simulink model "DFIG_WT_MPC"  (R2018a)
settings: Solver=VariableStepAuto  StartTime=0.0  StopTime=10.0  RelTol=1e-3
undefined symbols (not defined in the file): D1, Delta, powergui
libraries: powerlib x20, powerlib_meascontrol x18, fl_lib x6, nesl_utility x3, sdl_lib x1, simulink x1, re_lib x1
settings Model: Creator=Consultotal  LastModifiedBy=Consultotal
settings DebuggingCC: LibraryContextMissingDiagnostic=warning
settings SFSimCC: SimUseLocalCustomCode=on
settings RTWCC: RTWUseLocalCustomCode=on

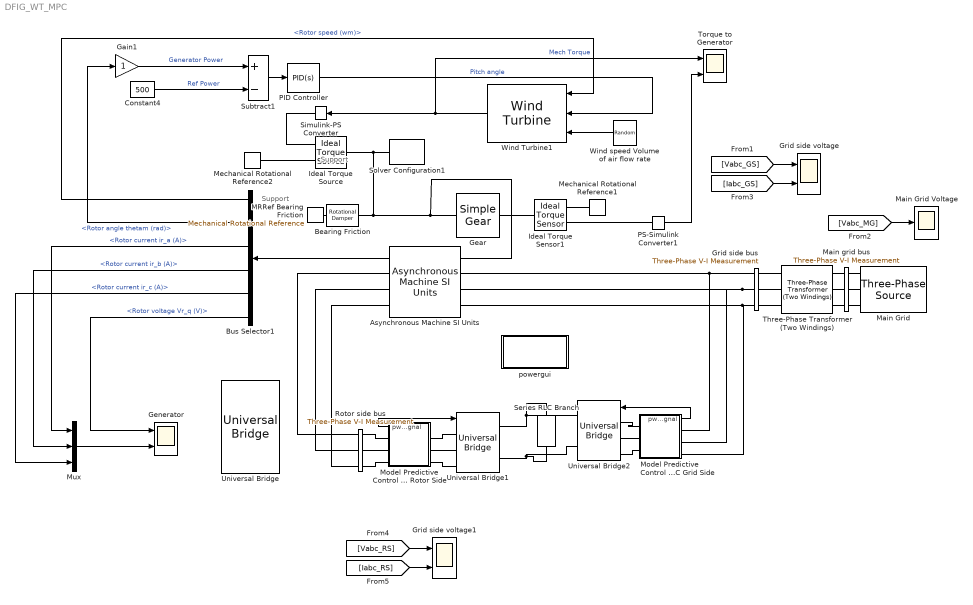
== system DFIG_WT_MPC ==
  note: Support
  note: Support
  Asynchronous Machine SI Units : powerlib/Machines/Asynchronous Machine SI Units  RotorType=Wound  PresetModel=No  MechanicalLoad=Mechanical rotational port  ShowDetailedParameters=on  ReferenceFrame=Synchronous  Units=SI  MeasurementBus=off  NominalParameters=[750e3 220 50]  Stator=[0.5968 0.0003495]  Rotor=[0.6258 0.005473]  Cage1=[0.4155 0.002066]  Cage2=[0.4168 0.0003495]  Lm=0.0354  Mechanical=[0.05 0.005879 2]  PolePairs=2  InitialConditions=[0 0 0 0 0 0 0 0]  SimulateSaturation=off  Saturation=[14.03593122, 27.81365428, 53.79336849, 72.68890987, 97.98006896, 148.6815601, 215.7428561, 302.9841135, 428.7778367 ; 230, 322, 414, 460, 506, 552, 598, 644, 690]  LoadFlowParameters=1492000  TsPowergui=0  TsBlock=-1  IterativeModel=Trapezoidal non iterative  IterativeDiscreteModel=Trapezoidal non iterative  Pmec=1.492e+006
  Bearing Friction : fl_lib/Mechanical/Rotational Elements/Rotational Damper  D=0.002 N*m/(rad/s)  w_specify=off  w_priority=High  w=0 rad/s  w_nominal_specify=off  w_nominal_unit=rad/s  w_nominal_value=1  t_specify=off  t_priority=High  t=0 N*m  t_nominal_specify=off  t_nominal_unit=N*m  t_nominal_value=1
  Bus Selector1 : BusSelector  OutputSignals=Mechanical.Rotor speed (wm),Mechanical.Rotor angle thetam (rad),Rotor measurements.Rotor current ir_a (A),Rotor measurements.Rotor current ir_b (A),Rotor measurements.Rotor current ir_c (A),Rotor measurements.Rotor voltage Vr_q (V)
  Constant4 : Constant  Value=500
  Gain1 : Gain
  Gear : sdl_lib/Gears/Simple Gear  ratio=40  rotation_direction=1  friction_model=1  T_noload=0.01 N*m  T_nom=0.2 N*m  efficiency_nom=0.8  efficiency=0.8  mu_visc=[ 0 0 ] N*m/(rad/s)  w_thr=0.01 rad/s  pwr_thr=0.001 W  enable_faults=0  efficiency_fault=0.05  external_fault=simscape.enum.onoff.off  temporal_fault=0  fault_time=5 s  fault_angles=pi / 12 rad  report_fault=1  temperature_TLU=[ 280 300 320 ] K  load_TLU=[ 1 5 10 ] N*m  efficiency_TLU=[ 0.95 0.9 0.85 ]  efficiency_TLU2=[ 0.85 0.8 0.75; 0.95 0.9 0.85; 0.85 0.8 0.7 ]  thermal_mass=50 J/K  T_init=300 K
      settings: SourceProductName=Simscape Driveline
  Generator : Scope  NumInputPorts=2
  Grid side bus : powerlib/Measurements/Three-Phase V-I Measurement  VoltageMeasurement=phase-to-phase  SetLabelV=on  LabelV=Vabc_GS  Vpu=off  VpuLL=off  CurrentMeasurement=yes  SetLabelI=on  LabelI=Iabc_GS  Ipu=off  Pbase=100e6  Vbase=18e3  OutputType=Complex  PhasorSimulation=off  PSBequivalent=0
  Grid side voltage : Scope  NumInputPorts=2
  Grid side voltage1 : Scope  NumInputPorts=2
  Ideal Torque Sensor1 : fl_lib/Mechanical/Mechanical Sensors/Ideal Torque Sensor
  Ideal Torque Source : fl_lib/Mechanical/Mechanical Sources/Ideal Torque Source
  MRRef Bearing Friction : fl_lib/Mechanical/Rotational Elements/Mechanical Rotational Reference
  Main grid bus : powerlib/Measurements/Three-Phase V-I Measurement  VoltageMeasurement=phase-to-phase  SetLabelV=on  LabelV=Vabc_MG  Vpu=off  VpuLL=off  CurrentMeasurement=no  SetLabelI=on  LabelI=Iabc_ld  Ipu=off  Pbase=100e6  Vbase=18e3  OutputType=Complex  PhasorSimulation=off  PSBequivalent=0
  Main Grid : powerlib/Electrical Sources/Three-Phase Source  InternalConnection=Yg  VoltagePhases=off  Voltage=34.5e3  PhaseAngle=0  Voltage_phases=[25e3 25e3 25e3]/sqrt(3)  PhaseAngles_phases=[0 -120 +120]  Frequency=50  NonIdealSource=on  SpecifyImpedance=off  Resistance=0.8929  Inductance=16.58e-3  ShortCircuitLevel=100e6  BaseVoltage=25e3  XRratio=7  BusType=swing  Pref=10e3  Qref=0  Prefabc=[10e3, 10e3, 10e3]  Qrefabc=[0, 0, 0]  Qmin=-inf  Qmax=inf
  Main Grid Voltage : Scope
  Mechanical Rotational Reference1 : fl_lib/Mechanical/Rotational Elements/Mechanical Rotational Reference
  Mechanical Rotational Reference2 : fl_lib/Mechanical/Rotational Elements/Mechanical Rotational Reference
  Model Predictive Control MPC Grid Side : Subsystem
  Model Predictive Control MPC Rotor Side : Subsystem
  Mux : Mux  Inputs=3
  PID Controller : simulink/Continuous/PID Controller  Controller=PID  Form=Parallel  TimeDomain=Continuous-time  SampleTime=-1  IntegratorMethod=Forward Euler  FilterMethod=Forward Euler  ControllerParametersSource=internal  P=5  I=8  D=0  UseFilter=on  N=100  TunerSelectOption=Transfer Function Based (PID Tuner App)  InitialConditionSource=internal  InitialConditionForIntegrator=0  InitialConditionForFilter=0  DifferentiatorICPrevScaledInput=0  ExternalReset=none  TrackingMode=off  Kt=1  LimitOutput=off  UpperSaturationLimit=inf  LowerSaturationLimit=-inf  LinearizeAsGain=on  AntiWindupMode=none  Kb=1  POutMin=[]  POutMax=[]  IOutMin=[]  IOutMax=[]  DOutMin=[]  DOutMax=[]  NOutMin=[]  NOutMax=[]  SumOutMin=[]  SumOutMax=[]  SaturationOutMin=[]  SaturationOutMax=[]  PParamMin=[]  PParamMax=[]  IParamMin=[]  IParamMax=[]  DParamMin=[]  DParamMax=[]  NParamMin=[]  NParamMax=[]  KbParamMin=[]  KbParamMax=[]  KtParamMin=[]  KtParamMax=[]  KbOutMin=[]  KbOutMax=[]  KtOutMin=[]  KtOutMax=[]  IntegratorOutMin=[]  IntegratorOutMax=[]  FilterOutMin=[]  FilterOutMax=[]  SumI1OutMin=[]  SumI1OutMax=[]  SumI2OutMin=[]  SumI2OutMax=[]  SumI3OutMin=[]  SumI3OutMax=[]  SumDOutMin=[]  SumDOutMax=[]  DifferentiatorOutMin=[]  DifferentiatorOutMax=[]  FilterDiffOutCoefMin=[]  FilterDiffOutCoefMax=[]  ReciprocalOutMin=[]  ReciprocalOutMax=[]  SumDenOutMin=[]  SumDenOutMax=[]  SumNumOutMin=[]  SumNumOutMax=[]  DivideOutMin=[]  DivideOutMax=[]  IntegratorContinuousStateAttributes=''  IntegratorStateMustResolveToSignalObject=off  IntegratorRTWStateStorageClass=Auto  FilterContinuousStateAttributes=''  FilterStateMustResolveToSignalObject=off  FilterRTWStateStorageClass=Auto
  PS-Simulink Converter1 : nesl_utility/PS-Simulink Converter  PhysicalDomain=network_engine_domain  SubClassName=ps_output  LeftPortType=input  RightPortType=output  PseudoPeriodic=off  Frequencies=[]  Unit=1  AffineConversion=off
  Rotor side bus : powerlib/Measurements/Three-Phase V-I Measurement  VoltageMeasurement=phase-to-phase  SetLabelV=on  LabelV=Vabc_RS  Vpu=off  VpuLL=off  CurrentMeasurement=yes  SetLabelI=on  LabelI=Iabc_RS  Ipu=off  Pbase=100e6  Vbase=18e3  OutputType=Complex  PhasorSimulation=off  PSBequivalent=0
  Series RLC Branch : powerlib/Elements/Series RLC Branch  LConnTagsString=__new0  RConnTagsString=__new0  BranchType=C  Resistance=1  Inductance=1e-3  SetiL0=off  InitialCurrent=0  Capacitance=1e6  Setx0=off  InitialVoltage=0  Measurements=None
  Simulink-PS Converter : nesl_utility/Simulink-PS Converter  PhysicalDomain=network_engine_domain  SubClassName=ps_input  LeftPortType=input  RightPortType=output  PseudoPeriodic=off  Frequencies=[]  NoiseDistribution=none  NoiseParameters=[]  Unit=1  AffineConversion=off  FilteringAndDerivatives=provide  SimscapeFilterOrder=1  InputFilterTimeConstant=0.001  UdotUserProvided=0
  Solver Configuration1 : nesl_utility/Solver Configuration  PhysicalDomain=network_engine_domain  SubClassName=solver  LeftPortType=input  RightPortType=generic  Tones=[]  Harmonics=[]  SimulateNoise=off  Profile=off  UseLocalSampling=off  EnableSwitchedLinearOptims=on  FrequencyDomain=off  UseCCode=off  RelTol=0.001  AbsTol=1e-06  MinStep=1e-09  ToWorkspace=off  RevertToSquareIcSolve=off  NumHomotopyIterations=100  PhasorMode=off  PhasorModeNumHarmonics=1  DoDC=off  ResidualTolerance=1e-9  UseLocalSolver=on  LocalSolverChoice=NE_BACKWARD_EULER_ADVANCER  LocalSolverSampleTime=.001  DoFixedCost=on  MaxNonlinIter=3  MaxModeIter=2  LinearAlgebra=Sparse  EquationFormulation=NE_TIME_EF  DelaysMemoryBudget=1024  AutomaticFiltering=on  FilteringTimeConstant=0.001  PartitionStorageMethod=AS_NEEDED  PartitionMemoryBudget=1024
  Subtract1 : Sum  Inputs=+-
  Three-Phase Transformer (Two Windings) : powerlib/Elements/Three-Phase Transformer (Two Windings)  Winding1Connection=Yg  Winding2Connection=Delta (D1)  CoreType=Three single-phase transformers  SetSaturation=off  Hysteresis=off  DataFile='hysteresis'  SetInitialFlux=off  Measurements=None  UNITS=pu  NominalPower=[ 75e3 , 50 ]  Winding1=[ 220 , 0.002 , 0.08 ]  Winding2=[ 34.5e3 , 0.002 , 0.08 ]  Rm=1e4  Lm=1e4  L0=0.5  Saturation=[ 0,0 ; 0.0024,1.2 ; 1.0,1.52 ]  InitialFluxes=[ 0.8 , -0.8 , 0.7 ]  MoreParameters=off  BreakLoop=off  DataType=off  TransfoNumber=1
  "Torque to Generator " : Scope  NumInputPorts=2
  Universal Bridge : powerlib/Power Electronics/Universal Bridge  Arms=3  SnubberResistance=1e5  SnubberCapacitance=inf  Device=Thyristors  Ron=1e-3  Lon=0  ForwardVoltages="[  0  0  ]"  ForwardVoltage=0  GTOparameters=[ 10e-6 , 20e-6 ]  IGBTparameters=[ 1e-6 , 2e-6 ]  Measurements=None  Measurements_2=None  converterType=Rectifier
  Universal Bridge1 : powerlib/Power Electronics/Universal Bridge  Arms=3  SnubberResistance=1e5  SnubberCapacitance=inf  Device=MOSFET / Diodes  Ron=1e-3  Lon=0  ForwardVoltages="[  0  0  ]"  ForwardVoltage=0  GTOparameters=[ 10e-6 , 20e-6 ]  IGBTparameters=[ 1e-6 , 2e-6 ]  Measurements=None  Measurements_2=None  converterType=Rectifier
  Universal Bridge2 : powerlib/Power Electronics/Universal Bridge  Arms=3  SnubberResistance=1e5  SnubberCapacitance=inf  Device=MOSFET / Diodes  Ron=1e-3  Lon=0  ForwardVoltages="[  0  0  ]"  ForwardVoltage=0  GTOparameters=[ 10e-6 , 20e-6 ]  IGBTparameters=[ 1e-6 , 2e-6 ]  Measurements=None  Measurements_2=None  converterType=Rectifier
  Wind Turbine1 : re_lib/Wind Generation/Wind Turbine  Pnom=1.5e6  Pelec_base=1.5e6/0.9  wind_base=12  P_wind_base=0.73  speed_nom=1.2  pitch_angle=0  c1_c6="[0.51763          116          0.4            5           21     0.006795]"  cp_nom=0.48  lambda_nom=8.1
      settings: SourceProductName=Simscape Power Systems  SourceProductBaseCode=PS
  Wind speed Volume of air flow rate : UniformRandomNumber  Minimum=2  Maximum=9  Seed=14  SampleTime=0.001
  powergui : Subsystem  Priority=1  AncestorBlock=powerlib/powergui  DialogController=POWERSYS.PowerSysDialog  InitFcn=powergui( 'InitFcn_Callback' , gcb , 0 , [ ] );  mask(PSB option menu block){SimulationMode=Discrete, SampleTime=50e-6, frequency=60, Iterations=50, frequencyindice=0, Pbase=100e6, ErrMax=1e-4, UnitsV=kV, UnitsW=MW, buscounter=0, FunctionMessages=off, echomessages=off, EnableUseOfTLC=off, CurrentSourceSwitches=off, DisableSnubberDevices=off, DisableRonSwitches=off, DisableVfSwitches=off, DisplayEquations=off, SolverType=Tustin/Backward Euler (TBE), Interpol=off, ExternalGateDelay=off, methode=off, Ts=100, x0status=blocks, SPID=on, SwTol=0, HookPort=off, RestoreLinks=warning, ResistiveCurrentMeasurement=off, Frange=[0:2:500], Ylog=off, Xlog=on, ShowGrid=off, save=off, variable=ZData, structure=0, ZoomFFT=off, StartTime=0.0, cycles=1, DisplayStyle=1, fundamental=60, FreqAxis=off, MaxFrequency=1000, frequencyindicesteady=1, RmsSteady=1, display=off}
      mask prompts: SimulationMode "Simulation type:"; SampleTime "Sample time (s):"; frequency "Frequency (Hz):"; Iterations "Max iterations"; frequencyindice "Frequency (Hz)"; Pbase "Base power (VA)"; ErrMax "PQ tolerance (pu)"; UnitsV "Voltage units"; UnitsW "Power units"; buscounter "Load flow bus counter"; FunctionMessages "Disable Specialized Power Systems warnings"; echomessages "Display Specialized Power Systems compilation messages"; EnableUseOfTLC "Use TLC file when in Accelerator Simulation Mode and for code generation"; CurrentSourceSwitches "Disable ideal switching"; DisableSnubberDevices "Disable snubbers in switching devices"; DisableRonSwitches "Disable Ron resistances in switching devices"; DisableVfSwitches "Disable forward voltages in switching devices"; DisplayEquations "Display circuit differential equations"; SolverType "Discrete solver"; Interpol "Interpolate switching events"; ExternalGateDelay "Use time-stamped gate signals"; methode "Store switching topologies"; Ts "Buffer size (MBytes):"; x0status "Start simulation with initial electrical states from:"; SPID "Use ideal switching devices"; SwTol "Switch tolerance"; HookPort "Allow multiple powergui blocks"; RestoreLinks "Restore disabled links of Simscape Power Systems ST blocks:"; ResistiveCurrentMeasurement "Use non ideal current measurement blocks (1e-4Ohm internal resistance)"; Frange "Frequency Range"; Ylog "Log impedance"; Xlog "log Frequency"; ShowGrid "grid"; save "Save Data To Workspace"; variable "Variable Name"; structure "Structure Name (PSBFFTSCOPE)"; ZoomFFT "ZoomFFT (PSBFFTSCOPE)"; StartTime "Start Time (PSBFFTSCOPE)"; cycles "Cycles (PSBFFTSCOPE)"; DisplayStyle "Display style (PSBFFTSCOPE)"; fundamental "Fundamental (PSBFFTSCOPE)"; FreqAxis "Frequency Axis (PSBFFTSCOPE)"; MaxFrequency "Max Frequency (PSBFFTSCOPE)"; frequencyindicesteady "Frequency indice (STEADYSTATE)"; RmsSteady "RMS display (STEADYSTATE)"; display "Display Results"
      mask help: Set simulation type, simulation parameters, and preferences.
      mask init:
      | dispMessage = powergui('MaskInitialization',gcb,SimulationMode,SampleTime);
      settings: PreSaveFcn=powergui( 'PreSaveFcn_Callback' , gcb , [ ] , [ ] );  OpenFcn=sps_rtmsupport('OpenFcn',gcbh)
      mask Help: helpview(psbhelp)
      mask TypeOptions SimulationMode: Continuous | Discrete | Phasor
      mask Callback SimulationMode: powergui('SimulationType',[],[],gcb);
      mask TypeOptions UnitsV: V | kV
      mask TypeOptions UnitsW: W | kW | MW
      mask Callback CurrentSourceSwitches: powergui('SimulationType',[],[],gcb);
      mask TypeOptions SolverType: Tustin/Backward Euler (TBE) | Tustin | Backward Euler
      mask Callback SolverType: powergui('SimulationType',[],[],gcb);
      mask Callback Interpol: powergui('SimulationType',[],[],gcb);
      mask Callback ExternalGateDelay: powergui('SimulationType',[],[],gcb);
      mask Callback methode: powergui('SimulationType',[],[],gcb);
      mask TypeOptions x0status: blocks | steady | zero
      mask TypeOptions RestoreLinks: yes | warning | no
      mask Callback display: sps_rtmsupport('parametereditingmodes',gcbh) % Will be executed last in parameter callbacks to ensure mask enable consistency
      mask DialogControl SolverTab Prompt: Solver
      mask DialogControl AutoSolverNote Prompt: To enable the Powergui solver settings, unselect auto (Automatic solver selection) solver in the Simulink solver options.
      mask DialogControl AnalysisTools Prompt: Tools
      mask DialogControl SteadyState Prompt: Steady-State
      mask DialogControl SteadyState Callback: close_system(gcb); power_steadystate(bdroot(gcb),gcb);
      mask DialogControl InitialState Prompt: Initial State
      mask DialogControl InitialState Callback: close_system(gcb); power_initstates(bdroot(gcb),gcb)
      mask DialogControl MachineInitialization Prompt: Machine Initialization
      mask DialogControl MachineInitialization Callback: close_system(gcb); power_loadflow(bdroot(gcb),gcb);
      mask DialogControl ImpedanceMeasurement Prompt: Impedance Measurement
      mask DialogControl ImpedanceMeasurement Callback: close_system(gcb); power_zmeter(bdroot(gcb),gcb);
      mask DialogControl FFTAnalysis Prompt: FFT Analysis
      mask DialogControl FFTAnalysis Callback: close_system(gcb); power_fftscope(bdroot(gcb),gcb);
      mask DialogControl LinearSystemAnalyzer Prompt: Use Linear System Analyzer
      mask DialogControl LinearSystemAnalyzer Callback: close_system(gcb); power_ltiview(bdroot(gcb),gcb);
      mask DialogControl HysteresisDesign Prompt: Hysteresis Design
      mask DialogControl HysteresisDesign Callback: close_system(gcb); power_hysteresis(bdroot(gcb),gcb);
      mask DialogControl RLCLineParameters Prompt: RLC Line Parameters
      mask DialogControl RLCLineParameters Callback: close_system(gcb); power_lineparam(bdroot(gcb),gcb);
      mask DialogControl GenerateReprot Prompt: Generate Report
      mask DialogControl GenerateReprot Callback: close_system(gcb); power_report(bdroot(gcb),gcb);
      mask DialogControl Control14 Prompt: Customize SPS blocks
      mask DialogControl Control14 Callback: close_system(gcb); power_customize;
      mask DialogControl LoadFlow Prompt: Load Flow
      mask DialogControl LoadFlow Callback: close_system(gcb); power_loadflow('-v2',bdroot(gcb));
      mask DialogControl Container14 Prompt: Load flow settings
      mask DialogControl ParameterTabVar012 Prompt: Preferences
      mask Display: color('blue'),disp(dispMessage)
  wires:
  PID Controller/1 -> Wind Turbine1/2  "Pitch angle"
  Subtract1/1 -> PID Controller/1
  Bus Selector1/1 -> Wind Turbine1/1  "<Rotor speed (wm)>"
  Bus Selector1/2 -> Gain1/1  "<Rotor angle thetam (rad)>"
  Wind Turbine1/1 -> Simulink-PS Converter/1, "Torque to Generator "/1  "Mech Torque"
  Constant4/1 -> Subtract1/2  "Ref Power"
  Gain1/1 -> Subtract1/1  "Generator Power"
  Wind speed Volume of air flow rate/1 -> Wind Turbine1/3
  Asynchronous Machine SI Units/1 -> Bus Selector1/1
  PS-Simulink Converter1/1 -> "Torque to Generator "/2
  Bus Selector1/6 -> Generator/1  "<Rotor voltage Vr_q (V)>"
  [Vabc_GS] -> Grid side voltage/1
  [Vabc_MG] -> Main Grid Voltage/1
  Mux/1 -> Generator/2
  Bus Selector1/3 -> Mux/1  "<Rotor current ir_a (A)>"
  Bus Selector1/4 -> Mux/2  "<Rotor current ir_b (A)>"
  Bus Selector1/5 -> Mux/3  "<Rotor current ir_c (A)>"
  Model Predictive Control MPC Grid Side/1(pwm signal) -> Universal Bridge2/1
  [Iabc_GS] -> Grid side voltage/2
  [Iabc_RS] -> Grid side voltage1/2
  [Vabc_RS] -> Grid side voltage1/1
  Model Predictive Control MPC Rotor Side/1(pwm signal) -> Universal Bridge1/1
  connections:
  Series RLC Branch/LConn1 -- Universal Bridge1/RConn1 -- Universal Bridge2/RConn1
  Series RLC Branch/RConn1 -- Universal Bridge2/RConn2 -- Universal Bridge1/RConn2
  Asynchronous Machine SI Units/RConn3 -- Rotor side bus/LConn3
  Ideal Torque Sensor1/LConn1 -- Gear/RConn1
  Mechanical Rotational Reference1/LConn1 -- Ideal Torque Sensor1/RConn1
  Ideal Torque Sensor1/RConn2 -- PS-Simulink Converter1/LConn1
  Simulink-PS Converter/RConn1 -- Ideal Torque Source/RConn1
  Ideal Torque Source/RConn2 -- Mechanical Rotational Reference2/LConn1
  Gear/LConn1 -- Asynchronous Machine SI Units/LConn1 -- Ideal Torque Source/LConn1 -- Solver Configuration1/RConn1 -- Bearing Friction/LConn1
  Rotor side bus/LConn2 -- Asynchronous Machine SI Units/RConn2
  Rotor side bus/LConn1 -- Asynchronous Machine SI Units/RConn1
  MRRef Bearing Friction/LConn1 -- Bearing Friction/RConn1
  Main Grid/RConn1 -- Main grid bus/RConn1
  Main grid bus/RConn2 -- Main Grid/RConn2
  Main Grid/RConn3 -- Main grid bus/RConn3
  Three-Phase Transformer (Two Windings)/RConn3 -- Main grid bus/LConn3
  Three-Phase Transformer (Two Windings)/RConn2 -- Main grid bus/LConn2
  Three-Phase Transformer (Two Windings)/RConn1 -- Main grid bus/LConn1
  Model Predictive Control MPC Grid Side/RConn1 -- Asynchronous Machine SI Units/LConn2 -- Grid side bus/LConn1
  Grid side bus/LConn2 -- Asynchronous Machine SI Units/LConn3 -- Model Predictive Control MPC Grid Side/RConn2
  Model Predictive Control MPC Grid Side/RConn3 -- Asynchronous Machine SI Units/LConn4 -- Grid side bus/LConn3
  Three-Phase Transformer (Two Windings)/LConn1 -- Grid side bus/RConn1
  Three-Phase Transformer (Two Windings)/LConn2 -- Grid side bus/RConn2
  Three-Phase Transformer (Two Windings)/LConn3 -- Grid side bus/RConn3
  Universal Bridge2/LConn1 -- Model Predictive Control MPC Grid Side/LConn1
  Universal Bridge2/LConn2 -- Model Predictive Control MPC Grid Side/LConn2
  Universal Bridge2/LConn3 -- Model Predictive Control MPC Grid Side/LConn3
  Model Predictive Control MPC Rotor Side/LConn2 -- Universal Bridge1/LConn1
  Universal Bridge1/LConn2 -- Model Predictive Control MPC Rotor Side/LConn3
  Model Predictive Control MPC Rotor Side/LConn4 -- Universal Bridge1/LConn3
  Model Predictive Control MPC Rotor Side/RConn3 -- Rotor side bus/RConn3
  Rotor side bus/RConn2 -- Model Predictive Control MPC Rotor Side/RConn2
  Rotor side bus/RConn1 -- Model Predictive Control MPC Rotor Side/RConn1

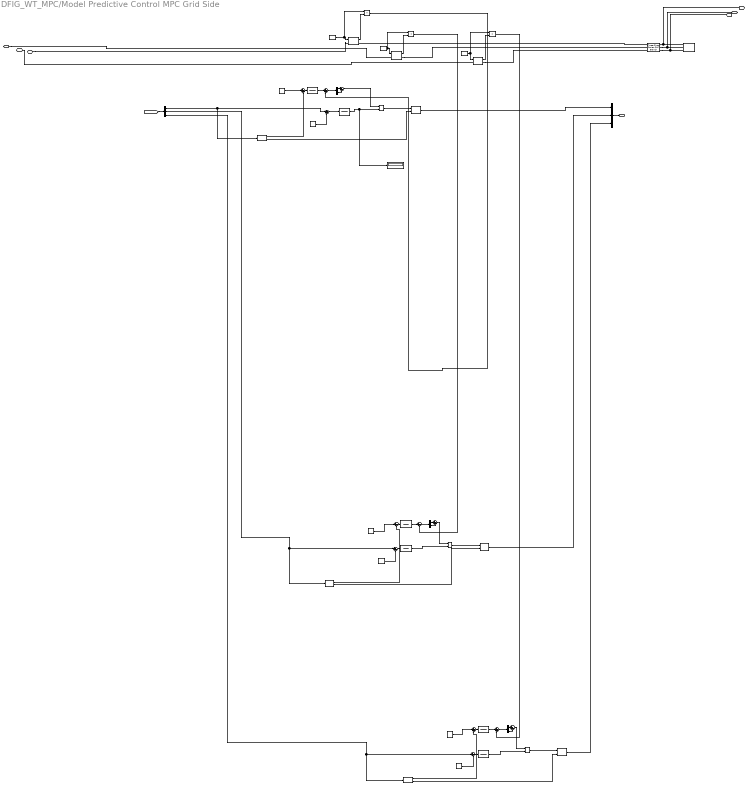
== system DFIG_WT_MPC/Model Predictive Control MPC Grid Side ==
  note: Amplitude of output voltage
  note: Delta ws
  note: deltaw
  note: wMG
  note: deltaE
  note: E*MG
  note: Fc= 50 Hz
  note: Amplitude of output voltage
  note: Delta ws
  note: deltaw
  note: wMG
  note: deltaE
  note: E*MG
  note: Fc= 50 Hz
  note: Amplitude of output voltage
  note: Delta ws
  note: deltaw
  note: wMG
  note: deltaE
  note: E*MG
  note: Fc= 50 Hz
  AC grid3 : powerlib/Elements/Three-Phase Series RLC Load  LConnTagsString=A|B|C  Configuration=Y (grounded)  NominalVoltage=240  Vabc=[1e3 1e3 1e3]  Vabcp=[1e3 1e3 1e3]  NominalFrequency=50  UnbalancedPower=off  ActivePower=10e4  InductivePower=0  CapacitivePower=0  Pabc=[10e3 9e3 11e3]  QLabc=[100 90 110]  QCabc=[100 90 110]  Pabcp=[10e3 9e3 11e3]  QLabcp=[100 90 110]  QCabcp=[100 90 110]  Measurements=None  LoadType=constant Z
  Demux : Demux  Outputs=3
  Demux1 : Demux  Outputs=2
  Demux3 : Demux  Outputs=2
  Demux4 : Demux  Outputs=2
  Discrete Transfer Fcn GE(S) : DiscreteTransferFcn  SampleTime=2e-6
  Discrete Transfer Fcn GE(S)1 : DiscreteTransferFcn  SampleTime=2e-6
  Discrete Transfer Fcn GE(S)2 : DiscreteTransferFcn  SampleTime=2e-6
  Discrete Transfer Fcn Gw(S) : DiscreteTransferFcn  SampleTime=2e-6
  Discrete Transfer Fcn Gw(S)1 : DiscreteTransferFcn  SampleTime=2e-6
  Discrete Transfer Fcn Gw(S)2 : DiscreteTransferFcn  SampleTime=2e-6
  Display1 : Display
  E*MG Amplitude's reference : Constant  Value=220
  E*MG Amplitude's reference1 : Constant  Value=220
  E*MG Amplitude's reference2 : Constant  Value=220
  Mux : Mux  Inputs=3
  PLL : powerlib_meascontrol/PLL/PLL  Fmin=45  Par_Init=[0, 50]  ParK=[0.45, 1.69, 0]  TcD=1e-4  MaxRateChangeFreq=12  FilterCutOffFreq=25  Ts=2e-6  AGC=on
      settings: SourceProductName=Simscape Power Systems  SourceProductBaseCode=PS
  PLL1 : powerlib_meascontrol/PLL/PLL  Fmin=45  Par_Init=[0, 50]  ParK=[0.45, 1.69, 0]  TcD=1e-4  MaxRateChangeFreq=12  FilterCutOffFreq=25  Ts=2e-6  AGC=on
      settings: SourceProductName=Simscape Power Systems  SourceProductBaseCode=PS
  PLL2 : powerlib_meascontrol/PLL/PLL  Fmin=45  Par_Init=[0, 50]  ParK=[0.45, 1.69, 0]  TcD=1e-4  MaxRateChangeFreq=12  FilterCutOffFreq=25  Ts=2e-6  AGC=on
      settings: SourceProductName=Simscape Power Systems  SourceProductBaseCode=PS
  PWM Generator (2-Level) : powerlib_meascontrol/Pulse & Signal Generators/PWM Generator (2-Level)  ModulatorType=Single-phase half-bridge (2 pulses)  ModulatorMode=Synchronized  Fc=27*50  Pc=90  nF=1  MinMax="[ -1  1 ]"  SamplingTechnique=Natural  ModulatingSignals=off  m=0.8  Freq=60  Phase=0  Ts=0  ShowCarrierOutport=off
      settings: SourceProductName=Simscape Power Systems
  PWM Generator (2-Level)1 : powerlib_meascontrol/Pulse & Signal Generators/PWM Generator (2-Level)  ModulatorType=Single-phase half-bridge (2 pulses)  ModulatorMode=Synchronized  Fc=27*50  Pc=90  nF=1  MinMax="[ -1  1 ]"  SamplingTechnique=Natural  ModulatingSignals=off  m=0.8  Freq=60  Phase=0  Ts=0  ShowCarrierOutport=off
      settings: SourceProductName=Simscape Power Systems
  PWM Generator (2-Level)2 : powerlib_meascontrol/Pulse & Signal Generators/PWM Generator (2-Level)  ModulatorType=Single-phase half-bridge (2 pulses)  ModulatorMode=Synchronized  Fc=27*50  Pc=90  nF=1  MinMax="[ -1  1 ]"  SamplingTechnique=Natural  ModulatingSignals=off  m=0.8  Freq=60  Phase=0  Ts=0  ShowCarrierOutport=off
      settings: SourceProductName=Simscape Power Systems
  Plant1 : powerlib/Elements/Three-Phase Series RLC Branch  LConnTagsString=A|B|C  RConnTagsString=A|B|C  BranchType=R  Resistance=0.05  Inductance=0.0002  Capacitance=0  Measurements=None
  Product1 : Product
  Product2 : Product
  Product3 : Product
  Product5 : Product  SampleTime=0  RndMeth=Zero
  Product7 : Product  SampleTime=0  RndMeth=Zero
  Product9 : Product  SampleTime=0  RndMeth=Zero
  Stair Generator : powerlib_meascontrol/Pulse & Signal Generators/Stair Generator  t="[0 3/60  8.25/60 ]"  e=[1 0 1]  Ts=0
      settings: SourceProductName=Simscape Power Systems
  Stair Generator1 : powerlib_meascontrol/Pulse & Signal Generators/Stair Generator  t="[0 3/60  8.25/60 ]"  e=[1 0 1]  Ts=0
      settings: SourceProductName=Simscape Power Systems
  Stair Generator2 : powerlib_meascontrol/Pulse & Signal Generators/Stair Generator  t="[0 3/60  8.25/60 ]"  e=[1 0 1]  Ts=0
      settings: SourceProductName=Simscape Power Systems
  Sum{4..6,9,11..13,16,19..21,24} (12 alike) : Sum  Inputs=|+-
  bypass : powerlib/Power Electronics/Ideal Switch  Ron=0.001  Lon=0  IC=0  Rs=1e5  Cs=inf  Measurements=on
  bypass1 : powerlib/Power Electronics/Ideal Switch  Ron=0.001  Lon=0  IC=0  Rs=1e5  Cs=inf  Measurements=on
  bypass2 : powerlib/Power Electronics/Ideal Switch  Ron=0.001  Lon=0  IC=0  Rs=1e5  Cs=inf  Measurements=on
  wi* island Frequency's reference : Constant  Value=50
  wi* island Frequency's reference1 : Constant  Value=50
  wi* island Frequency's reference2 : Constant  Value=50
  a : PMIOPort  Side=Right
  b : PMIOPort  Port=2  Side=Right
  c : PMIOPort  Port=3  Side=Right
  A : PMIOPort  Port=4  Side=Left
  B : PMIOPort  Port=5  Side=Left
  C : PMIOPort  Port=6  Side=Left
  pwm signal : Outport
  wires:
  Sum4/1 -> Discrete Transfer Fcn Gw(S)/1
  PLL1/2 -> PWM Generator (2-Level)1/2
  Discrete Transfer Fcn Gw(S)2/1 -> Sum20/1
  Demux/2 -> PLL1/1, Sum13/1
  Demux/3 -> PLL/1, Sum6/1
  bypass2/1 -> Product3/2
  Sum9/1 -> Product5/1
  Sum12/1 -> Demux3/1
  Sum11/1 -> Discrete Transfer Fcn Gw(S)1/1
  Demux3/1 -> Sum16/1
  E*MG Amplitude's reference1/1 -> Sum13/2
  PWM Generator (2-Level)2/1 -> Mux/1
  PWM Generator (2-Level)/1 -> Mux/3
  E*MG Amplitude's reference/1 -> Sum6/2
  PLL/2 -> PWM Generator (2-Level)/2
  Sum20/1 -> Demux4/1
  Stair Generator/1 -> bypass/1, Product2/1
  PLL2/1 -> Sum19/2
  wi* island Frequency's reference1/1 -> Sum11/1
  Stair Generator1/1 -> bypass1/1, Product1/1
  Discrete Transfer Fcn GE(S)1/1 -> Product7/2
  PLL2/2 -> PWM Generator (2-Level)2/2
  Product1/1 -> Sum12/2
  PLL1/1 -> Sum11/2
  E*MG Amplitude's reference2/1 -> Sum21/2
  Demux3/2 -> Sum16/2
  Product9/1 -> PWM Generator (2-Level)2/1
  Sum24/1 -> Product9/1
  Discrete Transfer Fcn Gw(S)/1 -> Sum5/1
  Product3/1 -> Sum5/2
  Discrete Transfer Fcn GE(S)2/1 -> Display1/1, Product9/2
  wi* island Frequency's reference2/1 -> Sum19/1
  Demux4/1 -> Sum24/1
  bypass/1 -> Product2/2
  Demux1/1 -> Sum9/1
  wi* island Frequency's reference/1 -> Sum4/1
  Sum19/1 -> Discrete Transfer Fcn Gw(S)2/1
  Demux1/2 -> Sum9/2
  bypass1/1 -> Product1/2
  Product2/1 -> Sum20/2
  Product5/1 -> PWM Generator (2-Level)/1
  Mux/1 -> pwm signal/1
  Sum6/1 -> Discrete Transfer Fcn GE(S)/1
  Discrete Transfer Fcn Gw(S)1/1 -> Sum12/1
  Sum13/1 -> Discrete Transfer Fcn GE(S)1/1
  Sum16/1 -> Product7/1
  PWM Generator (2-Level)1/1 -> Mux/2
  Demux4/2 -> Sum24/2
  Sum5/1 -> Demux1/1
  Discrete Transfer Fcn GE(S)/1 -> Product5/2
  Sum21/1 -> Discrete Transfer Fcn GE(S)2/1
  Demux/1 -> PLL2/1, Sum21/1
  Product7/1 -> PWM Generator (2-Level)1/1
  PLL/1 -> Sum4/2
  Stair Generator2/1 -> bypass2/1, Product3/1
  [Vabc_GS] -> Demux/1
  connections:
  C/RConn1 -- bypass/LConn1
  A/RConn1 -- bypass1/LConn1
  B/RConn1 -- bypass2/LConn1
  bypass2/RConn1 -- Plant1/RConn3
  bypass1/RConn1 -- Plant1/RConn2
  Plant1/RConn1 -- bypass/RConn1
  Plant1/LConn3 -- c/RConn1 -- AC grid3/LConn3
  Plant1/LConn2 -- b/RConn1 -- AC grid3/LConn2
  Plant1/LConn1 -- a/RConn1 -- AC grid3/LConn1

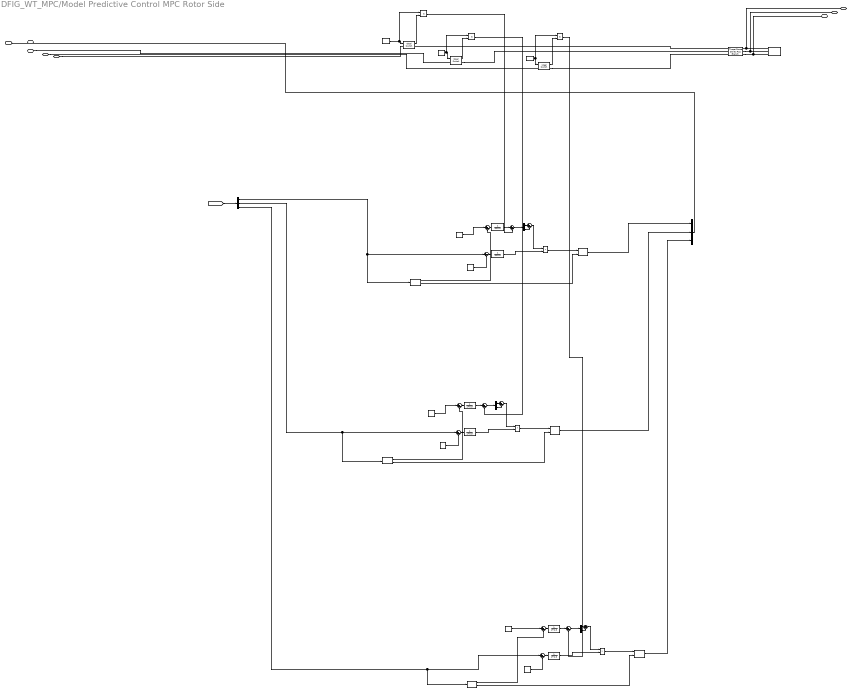
== system DFIG_WT_MPC/Model Predictive Control MPC Rotor Side ==
  note: Amplitude of output voltage
  note: Delta ws
  note: deltaw
  note: wMG
  note: deltaE
  note: E*MG
  note: Fc= 50 Hz
  note: Amplitude of output voltage
  note: Delta ws
  note: deltaw
  note: wMG
  note: deltaE
  note: E*MG
  note: Fc= 50 Hz
  note: Amplitude of output voltage
  note: Delta ws
  note: deltaw
  note: wMG
  note: deltaE
  note: E*MG
  note: Fc= 50 Hz
  AC grid3 : powerlib/Elements/Three-Phase Series RLC Load  LConnTagsString=A|B|C  Configuration=Y (grounded)  NominalVoltage=240  Vabc=[1e3 1e3 1e3]  Vabcp=[1e3 1e3 1e3]  NominalFrequency=50  UnbalancedPower=off  ActivePower=10e4  InductivePower=0  CapacitivePower=0  Pabc=[10e3 9e3 11e3]  QLabc=[100 90 110]  QCabc=[100 90 110]  Pabcp=[10e3 9e3 11e3]  QLabcp=[100 90 110]  QCabcp=[100 90 110]  Measurements=None  LoadType=constant Z
  Demux : Demux  Outputs=3
  Demux1 : Demux  Outputs=2
  Demux3 : Demux  Outputs=2
  Demux4 : Demux  Outputs=2
  Discrete Transfer Fcn GE(S) : DiscreteTransferFcn  SampleTime=2e-6
  Discrete Transfer Fcn GE(S)1 : DiscreteTransferFcn  SampleTime=2e-6
  Discrete Transfer Fcn GE(S)2 : DiscreteTransferFcn  SampleTime=2e-6
  Discrete Transfer Fcn Gw(S) : DiscreteTransferFcn  SampleTime=2e-6
  Discrete Transfer Fcn Gw(S)1 : DiscreteTransferFcn  SampleTime=2e-6
  Discrete Transfer Fcn Gw(S)2 : DiscreteTransferFcn  SampleTime=2e-6
  E*MG Amplitude's reference : Constant  Value=220
  E*MG Amplitude's reference1 : Constant  Value=220
  E*MG Amplitude's reference2 : Constant  Value=220
  Mux : Mux  Inputs=3
  PLL : powerlib_meascontrol/PLL/PLL  Fmin=45  Par_Init=[0, 50]  ParK=[0.45, 1.69, 0]  TcD=1e-4  MaxRateChangeFreq=12  FilterCutOffFreq=25  Ts=2e-6  AGC=on
      settings: SourceProductName=Simscape Power Systems  SourceProductBaseCode=PS
  PLL1 : powerlib_meascontrol/PLL/PLL  Fmin=45  Par_Init=[0, 50]  ParK=[0.45, 1.69, 0]  TcD=1e-4  MaxRateChangeFreq=12  FilterCutOffFreq=25  Ts=2e-6  AGC=on
      settings: SourceProductName=Simscape Power Systems  SourceProductBaseCode=PS
  PLL2 : powerlib_meascontrol/PLL/PLL  Fmin=45  Par_Init=[0, 50]  ParK=[0.45, 1.69, 0]  TcD=1e-4  MaxRateChangeFreq=12  FilterCutOffFreq=25  Ts=2e-6  AGC=on
      settings: SourceProductName=Simscape Power Systems  SourceProductBaseCode=PS
  PWM Generator (2-Level) : powerlib_meascontrol/Pulse & Signal Generators/PWM Generator (2-Level)  ModulatorType=Single-phase half-bridge (2 pulses)  ModulatorMode=Synchronized  Fc=27*50  Pc=90  nF=1  MinMax="[ -1  1 ]"  SamplingTechnique=Natural  ModulatingSignals=off  m=0.8  Freq=60  Phase=0  Ts=0  ShowCarrierOutport=off
      settings: SourceProductName=Simscape Power Systems
  PWM Generator (2-Level)1 : powerlib_meascontrol/Pulse & Signal Generators/PWM Generator (2-Level)  ModulatorType=Single-phase half-bridge (2 pulses)  ModulatorMode=Synchronized  Fc=27*50  Pc=90  nF=1  MinMax="[ -1  1 ]"  SamplingTechnique=Natural  ModulatingSignals=off  m=0.8  Freq=60  Phase=0  Ts=0  ShowCarrierOutport=off
      settings: SourceProductName=Simscape Power Systems
  PWM Generator (2-Level)2 : powerlib_meascontrol/Pulse & Signal Generators/PWM Generator (2-Level)  ModulatorType=Single-phase half-bridge (2 pulses)  ModulatorMode=Synchronized  Fc=27*50  Pc=90  nF=1  MinMax="[ -1  1 ]"  SamplingTechnique=Natural  ModulatingSignals=off  m=0.8  Freq=60  Phase=0  Ts=0  ShowCarrierOutport=off
      settings: SourceProductName=Simscape Power Systems
  Plant1 : powerlib/Elements/Three-Phase Series RLC Branch  LConnTagsString=A|B|C  RConnTagsString=A|B|C  BranchType=R  Resistance=0.05  Inductance=0.0002  Capacitance=0  Measurements=None
  Product1 : Product
  Product2 : Product
  Product3 : Product
  Product5 : Product  SampleTime=0  RndMeth=Zero
  Product7 : Product  SampleTime=0  RndMeth=Zero
  Product9 : Product  SampleTime=0  RndMeth=Zero
  Stair Generator : powerlib_meascontrol/Pulse & Signal Generators/Stair Generator  t="[0 3/60  8.25/60 ]"  e=[1 0 1]  Ts=0
      settings: SourceProductName=Simscape Power Systems
  Stair Generator1 : powerlib_meascontrol/Pulse & Signal Generators/Stair Generator  t="[0 3/60  8.25/60 ]"  e=[1 0 1]  Ts=0
      settings: SourceProductName=Simscape Power Systems
  Stair Generator2 : powerlib_meascontrol/Pulse & Signal Generators/Stair Generator  t="[0 3/60  8.25/60 ]"  e=[1 0 1]  Ts=0
      settings: SourceProductName=Simscape Power Systems
  Sum{4..6,9,11..13,16,19..21,24} (12 alike) : Sum  Inputs=|+-
  bypass : powerlib/Power Electronics/Ideal Switch  Ron=0.001  Lon=0  IC=0  Rs=1e5  Cs=inf  Measurements=on
  bypass1 : powerlib/Power Electronics/Ideal Switch  Ron=0.001  Lon=0  IC=0  Rs=1e5  Cs=inf  Measurements=on
  bypass2 : powerlib/Power Electronics/Ideal Switch  Ron=0.001  Lon=0  IC=0  Rs=1e5  Cs=inf  Measurements=on
  wi* island Frequency's reference : Constant  Value=50
  wi* island Frequency's reference1 : Constant  Value=50
  wi* island Frequency's reference2 : Constant  Value=50
  a : PMIOPort  Side=Right
  b : PMIOPort  Port=2  Side=Right
  c : PMIOPort  Port=3  Side=Right
  A1 : PMIOPort  Port=4  Side=Left
  A : PMIOPort  Port=5  Side=Left
  B : PMIOPort  Port=6  Side=Left
  C : PMIOPort  Port=7  Side=Left
  pwm signal : Outport
  wires:
  Sum4/1 -> Discrete Transfer Fcn Gw(S)/1
  PLL1/2 -> PWM Generator (2-Level)1/2
  Discrete Transfer Fcn Gw(S)2/1 -> Sum20/1
  Demux/2 -> PLL1/1, Sum13/1
  Demux/3 -> Sum6/1, PLL/1
  bypass2/1 -> Product3/2
  Sum9/1 -> Product5/1
  Sum12/1 -> Demux3/1
  Sum11/1 -> Discrete Transfer Fcn Gw(S)1/1
  Demux3/1 -> Sum16/1
  E*MG Amplitude's reference1/1 -> Sum13/2
  PWM Generator (2-Level)2/1 -> Mux/1
  PWM Generator (2-Level)/1 -> Mux/3
  E*MG Amplitude's reference/1 -> Sum6/2
  PLL/2 -> PWM Generator (2-Level)/2
  Sum20/1 -> Demux4/1
  Stair Generator/1 -> bypass/1, Product2/1
  PLL2/1 -> Sum19/2
  wi* island Frequency's reference1/1 -> Sum11/1
  Stair Generator1/1 -> bypass1/1, Product1/1
  Discrete Transfer Fcn GE(S)1/1 -> Product7/2
  PLL2/2 -> PWM Generator (2-Level)2/2
  Product1/1 -> Sum12/2
  PLL1/1 -> Sum11/2
  E*MG Amplitude's reference2/1 -> Sum21/2
  Demux3/2 -> Sum16/2
  Product9/1 -> PWM Generator (2-Level)2/1
  Sum24/1 -> Product9/1
  Discrete Transfer Fcn Gw(S)/1 -> Sum5/1
  Product3/1 -> Sum5/2
  Discrete Transfer Fcn GE(S)2/1 -> Product9/2
  wi* island Frequency's reference2/1 -> Sum19/1
  Demux4/1 -> Sum24/1
  bypass/1 -> Product2/2
  Demux1/1 -> Sum9/1
  wi* island Frequency's reference/1 -> Sum4/1
  Sum19/1 -> Discrete Transfer Fcn Gw(S)2/1
  Demux1/2 -> Sum9/2
  bypass1/1 -> Product1/2
  Product2/1 -> Sum20/2
  Product5/1 -> PWM Generator (2-Level)/1
  Mux/1 -> pwm signal/1
  Sum6/1 -> Discrete Transfer Fcn GE(S)/1
  Discrete Transfer Fcn Gw(S)1/1 -> Sum12/1
  Sum13/1 -> Discrete Transfer Fcn GE(S)1/1
  Sum16/1 -> Product7/1
  PWM Generator (2-Level)1/1 -> Mux/2
  Demux4/2 -> Sum24/2
  Sum5/1 -> Demux1/1
  Discrete Transfer Fcn GE(S)/1 -> Product5/2
  Sum21/1 -> Discrete Transfer Fcn GE(S)2/1
  Demux/1 -> PLL2/1, Sum21/1
  Product7/1 -> PWM Generator (2-Level)1/1
  PLL/1 -> Sum4/2
  Stair Generator2/1 -> bypass2/1, Product3/1
  [Vabc_RS] -> Demux/1
  connections:
  C/RConn1 -- bypass/LConn1
  A/RConn1 -- bypass1/LConn1
  B/RConn1 -- bypass2/LConn1
  Plant1/LConn1 -- a/RConn1 -- AC grid3/LConn1
  bypass2/RConn1 -- Plant1/RConn3
  bypass1/RConn1 -- Plant1/RConn2
  Plant1/RConn1 -- bypass/RConn1
  Plant1/LConn2 -- b/RConn1 -- AC grid3/LConn2
  Plant1/LConn3 -- c/RConn1 -- AC grid3/LConn3

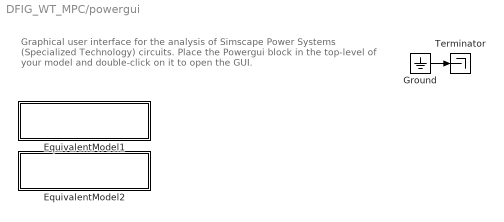
== system DFIG_WT_MPC/powergui ==
  note: Graphical user interface for the analysis of
      | Simscape Power Systems (Specialized Technology) circuits.
      | Place the Powergui block in the top-level of your model and double-click
      | on it to open the GUI.
  EquivalentModel1 : Subsystem
      mask init:
      | SPS = get_param(gcbh,'UserData');
      | if isempty(SPS)
      |     A=0;
      |     B=0;
      |     C=0;
      |     D=0;
      |     x0=0;
      | else
      | 	A=SPS.A;
      |     B=SPS.B;
      |     C=SPS.C;
      |     D=SPS.D;
      |     x0=SPS.x0;
      | end
      mask Display: disp('Dummy From Goto')
  EquivalentModel2 : Subsystem
      mask init:
      | S  = GetDataForEquivalentModel('Discrete',gcbh);
      mask Display:
      | color('red')
      | disp('EQUIVALENT CIRCUIT\nDiscrete')
  Ground : Ground
  Terminator : Terminator
  wires:
  Ground/1 -> Terminator/1

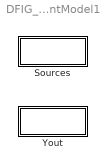
== system DFIG_WT_MPC/powergui/EquivalentModel1 ==
  Sources : Subsystem
  Yout : Subsystem

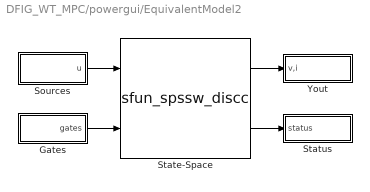
== system DFIG_WT_MPC/powergui/EquivalentModel2 ==
  Gates : Subsystem
  Sources : Subsystem
  State-Space : S-Function  FunctionName=sfun_spssw_discc  Parameters=S.Ts,S.A, S.B, S.C, S.D, S.x0, S.EnableUseOfTLC,S.SwitchResistance ,S.SwitchType, S.SwitchGateInitialValue, S.OutputsToResetToZero, S.TBEON,S.SaveMatrices,S.BufferSize  SFunctionDeploymentMode=off  EnableBusSupport=off
  Status : Subsystem
  Yout : Subsystem
  wires:
  Gates/1(gates) -> State-Space/2
  Sources/1(u) -> State-Space/1
  State-Space/2 -> Status/1(status)
  State-Space/1 -> Yout/1(v,i)

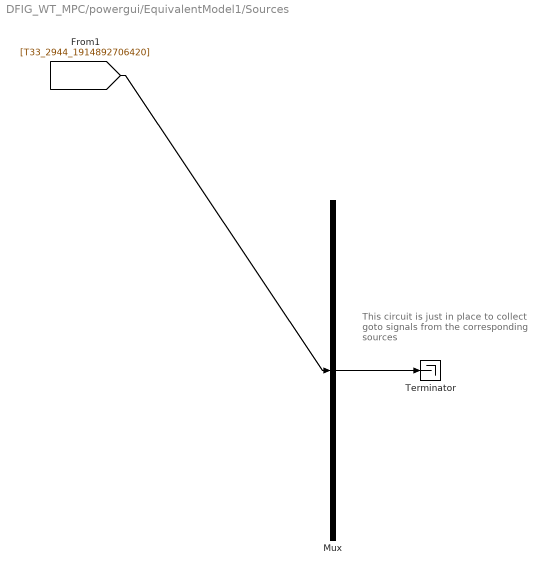
== system DFIG_WT_MPC/powergui/EquivalentModel1/Sources ==
  note: This circuit is just in place to collect
      | goto signals from the
      | corresponding sources
  Mux : Mux  Inputs=1
  Terminator : Terminator
  wires:
  Mux/1 -> Terminator/1
  [T33_2944_1914892706420] -> Mux/1

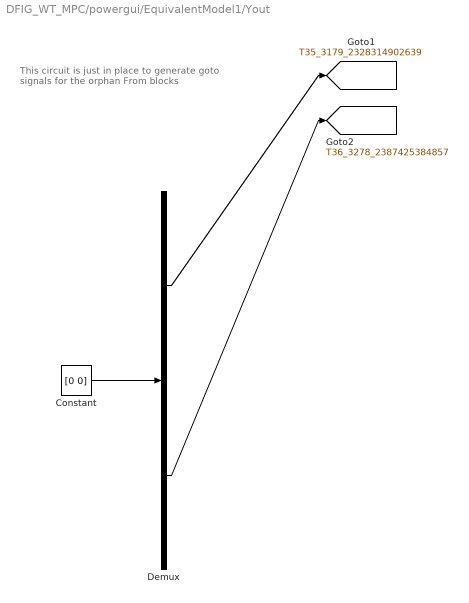
== system DFIG_WT_MPC/powergui/EquivalentModel1/Yout ==
  note: This circuit is just in place to generate
      | goto signals for the orphan From blocks
  Constant : Constant  Value=[0 0]
  Demux : Demux  Outputs=[1 1]
  tag scope: T35_3179_2328314902639=global, T36_3278_2387425384857=global
  wires:
  Constant/1 -> Demux/1
  Demux/1 -> [T35_3179_2328314902639]
  Demux/2 -> [T36_3278_2387425384857]

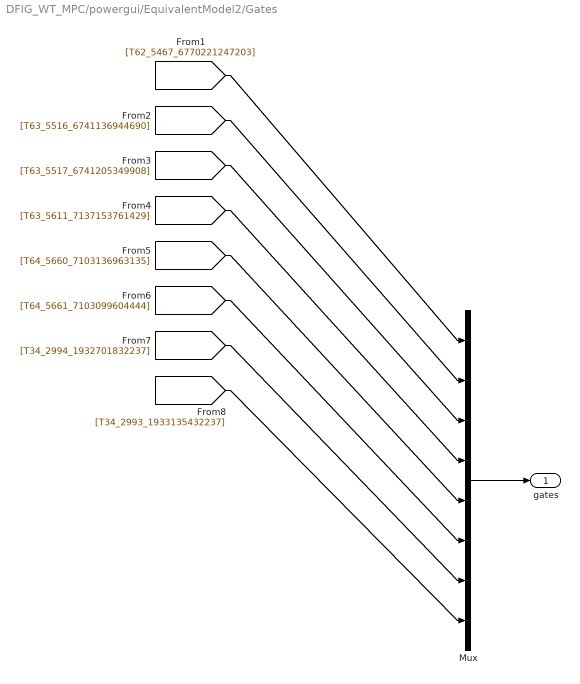
== system DFIG_WT_MPC/powergui/EquivalentModel2/Gates ==
  Mux : Mux  Inputs=[1 1 1 1 1 1 6 6]
  gates : Outport
  wires:
  Mux/1 -> gates/1
  [T62_5467_6770221247203] -> Mux/1
  [T63_5516_6741136944690] -> Mux/2
  [T63_5517_6741205349908] -> Mux/3
  [T63_5611_7137153761429] -> Mux/4
  [T64_5660_7103136963135] -> Mux/5
  [T64_5661_7103099604444] -> Mux/6
  [T34_2994_1932701832237] -> Mux/7
  [T34_2993_1933135432237] -> Mux/8

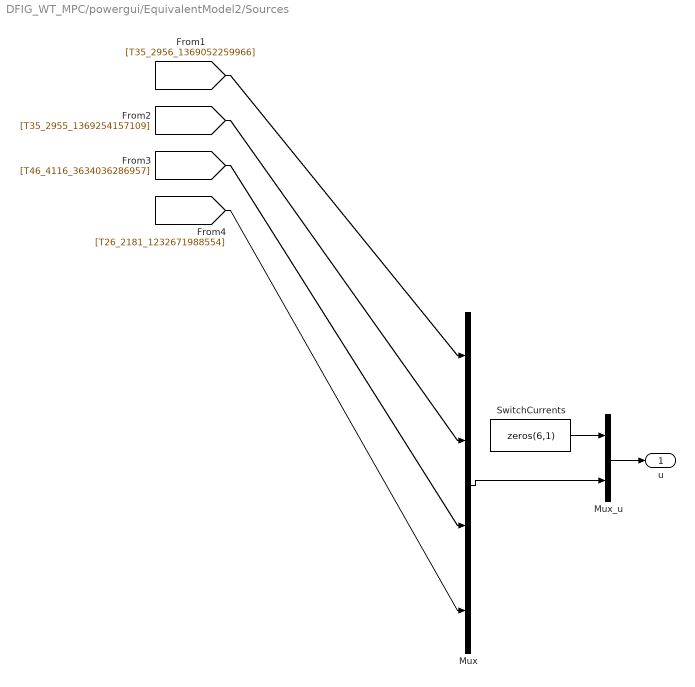
== system DFIG_WT_MPC/powergui/EquivalentModel2/Sources ==
  Mux : Mux  Inputs=[6 6 4 3]
  Mux_u : Mux  Inputs=[6 19]
  SwitchCurrents : Constant  Value=zeros(6,1)
  u : Outport
  wires:
  Mux_u/1 -> u/1
  SwitchCurrents/1 -> Mux_u/1
  Mux/1 -> Mux_u/2
  [T35_2956_1369052259966] -> Mux/1
  [T35_2955_1369254157109] -> Mux/2
  [T46_4116_3634036286957] -> Mux/3
  [T26_2181_1232671988554] -> Mux/4

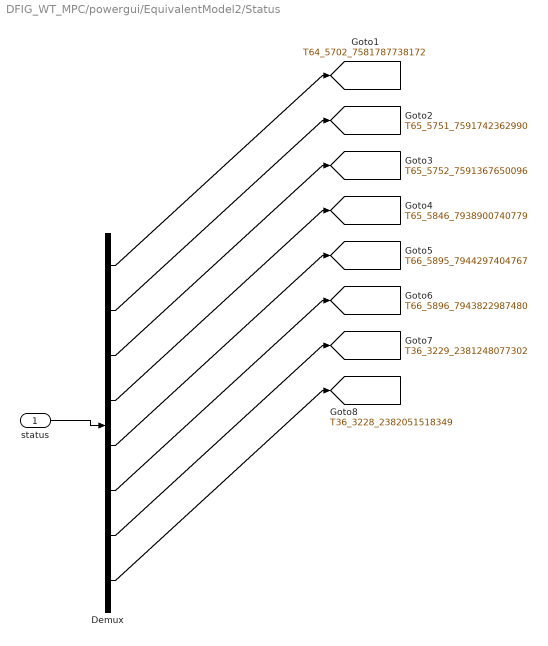
== system DFIG_WT_MPC/powergui/EquivalentModel2/Status ==
  status : Inport
  Demux : Demux  Outputs=[1 1 1 1 1 1 6 6]
  tag scope: T36_3228_2382051518349=global, T36_3229_2381248077302=global, T64_5702_7581787738172=global, T65_5751_7591742362990=global, T65_5752_7591367650096=global, T65_5846_7938900740779=global, T66_5895_7944297404767=global, T66_5896_7943822987480=global
  wires:
  status/1 -> Demux/1
  Demux/1 -> [T64_5702_7581787738172]
  Demux/2 -> [T65_5751_7591742362990]
  Demux/3 -> [T65_5752_7591367650096]
  Demux/4 -> [T65_5846_7938900740779]
  Demux/5 -> [T66_5895_7944297404767]
  Demux/6 -> [T66_5896_7943822987480]
  Demux/7 -> [T36_3229_2381248077302]
  Demux/8 -> [T36_3228_2382051518349]

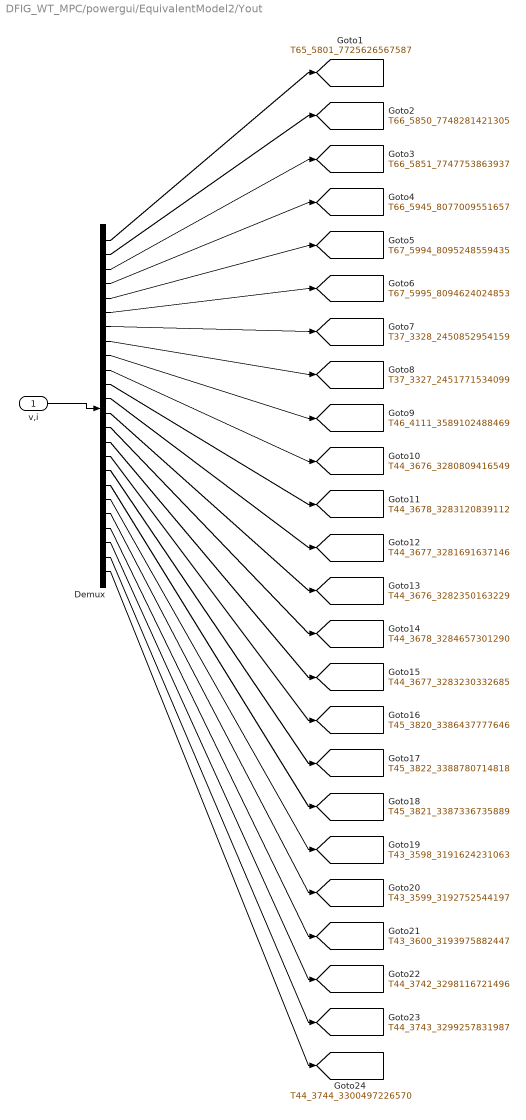
== system DFIG_WT_MPC/powergui/EquivalentModel2/Yout ==
  v,i : Inport
  Demux : Demux  Outputs=[1 1 1 1 1 1 6 6 4 1 1 1 1 1 1 1 1 1 1 1 1 1 1 1]
  tag scope: T37_3327_2451771534099=global, T37_3328_2450852954159=global, T43_3598_3191624231063=global, T43_3599_3192752544197=global, T43_3600_3193975882447=global, T44_3676_3280809416549=global, T44_3676_3282350163229=global, T44_3677_3281691637146=global, T44_3677_3283230332685=global, T44_3678_3283120839112=global, T44_3678_3284657301290=global, T44_3742_3298116721496=global, T44_3743_3299257831987=global, T44_3744_3300497226570=global, T45_3820_3386437777646=global, T45_3821_3387336735889=global, T45_3822_3388780714818=global, T46_4111_3589102488469=global, T65_5801_7725626567587=global, T66_5850_7748281421305=global, T66_5851_7747753863937=global, T66_5945_8077009551657=global, T67_5994_8095248559435=global, T67_5995_8094624024853=global
  wires:
  v,i/1 -> Demux/1
  Demux/1 -> [T65_5801_7725626567587]
  Demux/2 -> [T66_5850_7748281421305]
  Demux/3 -> [T66_5851_7747753863937]
  Demux/4 -> [T66_5945_8077009551657]
  Demux/5 -> [T67_5994_8095248559435]
  Demux/6 -> [T67_5995_8094624024853]
  Demux/7 -> [T37_3328_2450852954159]
  Demux/8 -> [T37_3327_2451771534099]
  Demux/9 -> [T46_4111_3589102488469]
  Demux/10 -> [T44_3676_3280809416549]
  Demux/11 -> [T44_3678_3283120839112]
  Demux/12 -> [T44_3677_3281691637146]
  Demux/13 -> [T44_3676_3282350163229]
  Demux/14 -> [T44_3678_3284657301290]
  Demux/15 -> [T44_3677_3283230332685]
  Demux/16 -> [T45_3820_3386437777646]
  Demux/17 -> [T45_3822_3388780714818]
  Demux/18 -> [T45_3821_3387336735889]
  Demux/19 -> [T43_3598_3191624231063]
  Demux/20 -> [T43_3599_3192752544197]
  Demux/21 -> [T43_3600_3193975882447]
  Demux/22 -> [T44_3742_3298116721496]
  Demux/23 -> [T44_3743_3299257831987]
  Demux/24 -> [T44_3744_3300497226570]
